simulink model "sampleModel1785_3_sub_sub"  (R2023a)
settings: Solver=VariableStepAuto  StartTime=0.0  StopTime=10.0  RelTol=1e-3
libraries: hdlsllib x4, simulink x2
settings Model: Creator=user1  LastModifiedBy=user1
settings OptimizationCC: BlockReduction=off  ConditionallyExecuteInputs=off

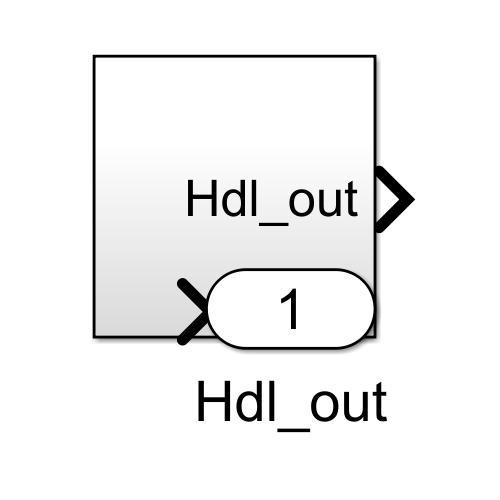
[thumbnail: Simulink's stored preview of the top-level diagram]
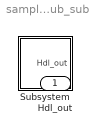
== system sampleModel1785_3_sub_sub ==
  Subsystem : Subsystem
  Hdl_out : Outport  OutDataTypeStr=uint8

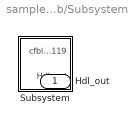
== system sampleModel1785_3_sub_sub/Subsystem ==
  Subsystem : Subsystem
  Hdl_out : Outport  OutDataTypeStr=uint8

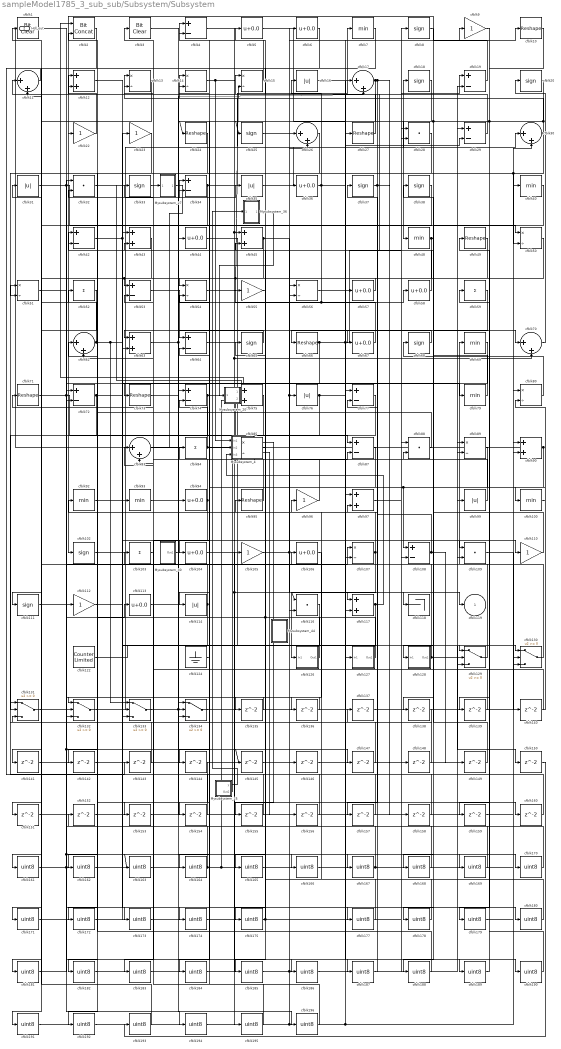
== system sampleModel1785_3_sub_sub/Subsystem/Subsystem ==
  Mysubsystem_20 : Subsystem  TreatAsAtomicUnit=on  RTWFcnName=Mysubsystem_20
      settings: RTWFcnNameOpts=User specified  RTWFileNameOpts=Use function name
  Mysubsystem_25 : Subsystem  TreatAsAtomicUnit=on  RTWFcnName=Mysubsystem_25
      settings: RTWFcnNameOpts=User specified  RTWFileNameOpts=Use function name
  Mysubsystem_27 : Subsystem  TreatAsAtomicUnit=on  RTWFcnName=Mysubsystem_27
      settings: RTWFcnNameOpts=User specified  RTWFileNameOpts=Use function name
  Mysubsystem_30 : Subsystem  TreatAsAtomicUnit=on  RTWFcnName=Mysubsystem_30
      settings: RTWFcnNameOpts=User specified  RTWFileNameOpts=Use function name
  Mysubsystem_36 : Subsystem  TreatAsAtomicUnit=on  RTWFcnName=Mysubsystem_36
      settings: RTWFcnNameOpts=User specified  RTWFileNameOpts=Use function name
  Mysubsystem_4 : Subsystem  TreatAsAtomicUnit=on  RTWFcnName=Mysubsystem_4
      settings: RTWFcnNameOpts=User specified  RTWFileNameOpts=Use function name
  Mysubsystem_44 : Subsystem  TreatAsAtomicUnit=on  RTWFcnName=Mysubsystem_44
      settings: RTWFcnNameOpts=User specified  RTWFileNameOpts=Use function name
  cfblk1 : simulink/Logic and Bit Operations/Bit Clear  iBit=0
      settings: LibrarySourceBlock=|
      | hdlsllib/Logic and Bit
      | Operations/Bit Clear
  cfblk{10,24,27,49,66,71,73,95} (8 alike) : Reshape
  cfblk{7,40,48,69,79,92..93,100} (8 alike) : MinMax  OutDataTypeStr=uint8
  cfblk{8,18,20,25,33,37..38,65,68,102,111} (11 alike) : Signum
  cfblk{52,59,84,103} (4 alike) : Sum  Inputs=+  OutDataTypeStr=uint8
  cfblk{5..6,36,44,57..58,67,94,104,106,113} (11 alike) : Bias  Bias=0.0  SaturateOnIntegerOverflow=off
  cfblk{9,22..23,55,96,105,110,112} (8 alike) : Gain  OutDataTypeStr=uint8
  cfblk{13..15,50..51,54,56,80,85,89,107} (11 alike) : Product  Inputs=*/  OutDataTypeStr=uint8  RndMeth=Zero  SaturateOnIntegerOverflow=on
  cfblk{4,19,29,34,42,53,64,72,74,77,87,108} (12 alike) : Sum  Inputs=+-  OutDataTypeStr=uint8
  cfblk{28,32,88,109,116} (5 alike) : DotProduct  OutDataTypeStr=uint8
  cfblk{11,17,26,30,62,70,83} (7 alike) : Sum  Inputs=|++  OutDataTypeStr=uint8
  cfblk{16,31,35,76,99,114} (6 alike) : Abs  OutDataTypeStr=uint8  SaturateOnIntegerOverflow=off
  cfblk{12,43,45,63,75,90,97,117} (8 alike) : Sum  OutDataTypeStr=uint8
  cfblk118 : Terminator
  cfblk122 : hdlsllib/Sources/Counter Limited  uplimit=7  tsamp=-1
  cfblk124 : Ground
  cfblk126 : Subsystem
      settings: LibrarySourceBlock=|
      | hdlsllib/Ports &
      | Subsystems/Subsystem
  cfblk127 : Subsystem
      settings: LibrarySourceBlock=|
      | hdlsllib/Ports &
      | Subsystems/Subsystem
  cfblk128 : Subsystem
      settings: LibrarySourceBlock=|
      | hdlsllib/Ports &
      | Subsystems/Subsystem
  cfblk{129..134} (6 alike) : Switch  OutDataTypeStr=uint8  SaturateOnIntegerOverflow=off  InputSameDT=off
  cfblk{135..160} (26 alike) : Delay  SampleTime=1
  cfblk{161..175,177..196} (35 alike) : DataTypeConversion  OutDataTypeStr=uint8  SaturateOnIntegerOverflow=off  RndMeth=Floor
  cfblk2 : hdlsllib/Logic and Bit Operations/Bit Concat  numInputs=2
  cfblk3 : simulink/Logic and Bit Operations/Bit Clear  iBit=0
      settings: LibrarySourceBlock=|
      | hdlsllib/Logic and Bit
      | Operations/Bit Clear
  cfblk119 : Outport  OutDataTypeStr=uint8  VectorParamsAs1DForOutWhenUnconnected=off
  Hdl_out : Outport  Port=2  OutDataTypeStr=uint8
  wires:
  Mysubsystem_36/1(Out1) -> Mysubsystem_20/1(In1)
  Mysubsystem_25/1(y) -> Mysubsystem_36/1(In1)
  Mysubsystem_30/1(Out1) -> cfblk134/3
  Mysubsystem_27/1(Out1) -> Mysubsystem_4/2(In2)
  Mysubsystem_20/2(Out2) -> Mysubsystem_27/1(In1)
  Mysubsystem_25/2(Out2) -> cfblk85/1
  Mysubsystem_20/1(Out1) -> cfblk2/1
  Mysubsystem_4/2(Out2) -> cfblk156/1
  Mysubsystem_4/1(Out1) -> cfblk155/1
  cfblk196/1 -> cfblk84/1
  cfblk3/1 -> cfblk196/1
  cfblk195/1 -> cfblk3/1
  cfblk54/1 -> cfblk195/1
  cfblk194/1 -> cfblk17/1, cfblk130/3, cfblk36/1
  cfblk193/1 -> cfblk1/1
  cfblk150/1 -> cfblk193/1
  cfblk192/1 -> cfblk56/2
  cfblk191/1 -> cfblk56/1
  cfblk52/1 -> cfblk191/1
  cfblk190/1 -> cfblk49/1
  cfblk56/1 -> cfblk190/1
  cfblk189/1 -> cfblk59/1
  cfblk188/1 -> cfblk152/1
  cfblk59/1 -> cfblk188/1
  cfblk187/1 -> cfblk77/2
  cfblk186/1 -> cfblk77/1
  cfblk185/1 -> cfblk146/1, cfblk109/2
  cfblk184/1 -> cfblk28/2
  cfblk183/1 -> cfblk28/1
  cfblk182/1 -> cfblk105/1
  cfblk28/1 -> cfblk182/1
  cfblk181/1 -> cfblk112/1
  cfblk13/1 -> cfblk181/1
  cfblk180/1 -> cfblk96/1
  cfblk112/1 -> cfblk180/1
  cfblk179/1 -> cfblk40/1
  cfblk9/1 -> cfblk179/1
  cfblk178/1 -> cfblk137/1
  cfblk40/1 -> cfblk178/1
  cfblk177/1 -> cfblk85/2
  cfblk12/1 -> cfblk177/1
  cfblk175/1 -> cfblk65/1, cfblk88/1
  cfblk174/1 -> cfblk26/2
  cfblk92/1 -> cfblk174/1
  cfblk173/1 -> cfblk26/1
  cfblk172/1 -> cfblk6/1
  cfblk26/1 -> cfblk172/1
  cfblk171/1 -> cfblk93/1
  cfblk170/1 -> cfblk89/1
  cfblk93/1 -> cfblk170/1
  cfblk169/1 -> cfblk83/2
  cfblk153/1 -> cfblk169/1
  cfblk168/1 -> cfblk83/1
  cfblk8/1 -> cfblk168/1
  cfblk167/1 -> cfblk32/1, cfblk29/1
  cfblk166/1 -> cfblk90/2
  cfblk32/1 -> cfblk166/1
  cfblk165/1 -> cfblk90/1
  cfblk55/1 -> cfblk165/1
  cfblk164/1 -> cfblk116/2, cfblk75/2, cfblk2/2
  cfblk163/1 -> cfblk43/2
  cfblk162/1 -> cfblk43/1
  cfblk144/1 -> cfblk162/1
  cfblk161/1 -> cfblk99/1, cfblk173/1
  cfblk160/1 -> cfblk54/2
  cfblk159/1 -> cfblk80/1
  cfblk10/1 -> cfblk159/1
  cfblk158/1 -> cfblk97/2
  cfblk157/1 -> cfblk14/2
  cfblk156/1 -> cfblk131/1
  cfblk155/1 -> cfblk72/1
  cfblk154/1 -> cfblk134/1
  cfblk87/1 -> cfblk154/1
  cfblk152/1 -> cfblk34/2
  cfblk151/1 -> cfblk30/2
  cfblk149/1 -> cfblk88/2
  cfblk148/1 -> cfblk12/2
  cfblk147/1 -> cfblk64/2
  cfblk146/1 -> cfblk19/2
  cfblk145/1 -> cfblk45/2
  cfblk116/1 -> cfblk144/1
  cfblk143/1 -> cfblk51/1
  cfblk11/1 -> cfblk143/1
  cfblk142/1 -> cfblk129/2
  cfblk75/1 -> cfblk142/1
  cfblk141/1 -> cfblk89/2
  cfblk6/1 -> cfblk141/1
  cfblk140/1 -> cfblk74/1
  cfblk109/1 -> cfblk140/1
  cfblk139/1 -> cfblk53/2
  cfblk138/1 -> cfblk131/3
  cfblk137/1 -> cfblk108/2
  cfblk136/1 -> cfblk132/2
  cfblk106/1 -> cfblk136/1
  cfblk135/1 -> cfblk132/1
  cfblk7/1 -> cfblk135/1
  cfblk29/1 -> cfblk12/1
  cfblk38/1 -> cfblk111/1
  cfblk30/1 -> cfblk50/2, cfblk114/1, cfblk24/1, cfblk13/2
  cfblk14/1 -> Mysubsystem_4/1(In1), cfblk45/1, cfblk129/3
  cfblk77/1 -> cfblk185/1
  cfblk4/1 -> cfblk70/2, cfblk109/1
  cfblk85/1 -> cfblk175/1
  cfblk20/1 -> cfblk25/1, cfblk138/1, cfblk139/1
  cfblk49/1 -> cfblk132/3, cfblk55/1
  cfblk107/1 -> cfblk126/1(In1), cfblk92/1
  cfblk42/1 -> cfblk23/1, cfblk147/1
  cfblk33/1 -> cfblk70/1
  cfblk24/1 -> cfblk63/2
  cfblk51/1 -> cfblk163/1, cfblk186/1, cfblk145/1
  cfblk73/1 -> cfblk35/1
  cfblk100/1 -> cfblk80/2
  cfblk95/1 -> cfblk62/2
  cfblk44/1 -> cfblk97/1
  cfblk58/1 -> cfblk13/1
  cfblk90/1 -> cfblk164/1, Hdl_out/1
  cfblk97/1 -> cfblk19/1
  cfblk63/1 -> cfblk94/1, cfblk17/2
  cfblk134/1 -> cfblk100/1
  cfblk50/1 -> cfblk53/1, cfblk151/1
  cfblk37/1 -> cfblk67/1, cfblk148/1
  cfblk62/1 -> cfblk110/1, cfblk133/1, cfblk11/2
  cfblk131/1 -> cfblk113/1
  cfblk23/1 -> cfblk51/2
  cfblk53/1 -> cfblk64/1
  cfblk124/1 -> cfblk4/2
  cfblk70/1 -> cfblk20/1
  cfblk15/1 -> cfblk4/1
  cfblk103/1 -> cfblk33/1
  cfblk88/1 -> cfblk52/1
  cfblk1/1 -> cfblk194/1
  cfblk68/1 -> cfblk66/1
  cfblk48/1 -> cfblk128/1(In1), cfblk171/1
  cfblk79/1 -> cfblk38/1
  cfblk65/1 -> cfblk63/1
  cfblk76/1 -> cfblk27/1, cfblk192/1
  cfblk45/1 -> cfblk76/1, cfblk117/2, cfblk104/1
  cfblk111/1 -> cfblk107/1
  cfblk128/1(Out1) -> cfblk103/1, cfblk150/1
  cfblk83/1 -> cfblk167/1
  cfblk72/1 -> cfblk130/2, cfblk131/2
  cfblk69/1 -> cfblk73/1
  cfblk94/1 -> cfblk71/1, cfblk183/1
  cfblk127/1(Out1) -> cfblk42/2, cfblk95/1
  cfblk57/1 -> cfblk54/1
  cfblk22/1 -> cfblk11/1
  cfblk122/1 -> cfblk130/1
  cfblk16/1 -> cfblk127/1(In1)
  cfblk2/1 -> cfblk22/1
  cfblk102/1 -> cfblk30/1
  cfblk114/1 -> cfblk31/1, cfblk153/1
  cfblk105/1 -> cfblk87/2, cfblk117/1
  cfblk31/1 -> cfblk50/1, cfblk189/1
  cfblk133/1 -> cfblk58/1, cfblk187/1
  cfblk84/1 -> cfblk116/1, cfblk160/1, cfblk74/2
  cfblk35/1 -> cfblk18/1
  cfblk104/1 -> cfblk118/1
  cfblk25/1 -> cfblk9/1
  cfblk67/1 -> cfblk15/2, cfblk16/1
  cfblk96/1 -> cfblk42/1
  cfblk99/1 -> cfblk75/1, cfblk32/2
  cfblk89/1 -> cfblk108/1, cfblk107/2
  cfblk71/1 -> cfblk87/1, cfblk79/1
  cfblk74/1 -> cfblk134/2, cfblk119/1
  cfblk17/1 -> cfblk157/1, cfblk158/1, cfblk184/1
  cfblk126/1(Out1) -> cfblk62/1
  cfblk117/1 -> Mysubsystem_4/3(In3), cfblk133/3
  cfblk5/1 -> cfblk57/1
  cfblk132/1 -> cfblk34/1
  cfblk80/1 -> cfblk68/1
  cfblk113/1 -> cfblk44/1
  cfblk27/1 -> cfblk5/1
  cfblk34/1 -> cfblk7/1, cfblk72/2
  cfblk129/1 -> cfblk69/1
  cfblk19/1 -> cfblk102/1
  cfblk36/1 -> cfblk14/1, cfblk29/2
  cfblk64/1 -> cfblk129/1
  cfblk66/1 -> cfblk8/1, cfblk10/1, cfblk133/2
  cfblk130/1 -> cfblk106/1
  cfblk110/1 -> cfblk15/1
  cfblk18/1 -> cfblk48/1
  cfblk43/1 -> cfblk161/1
  cfblk108/1 -> cfblk37/1, cfblk149/1

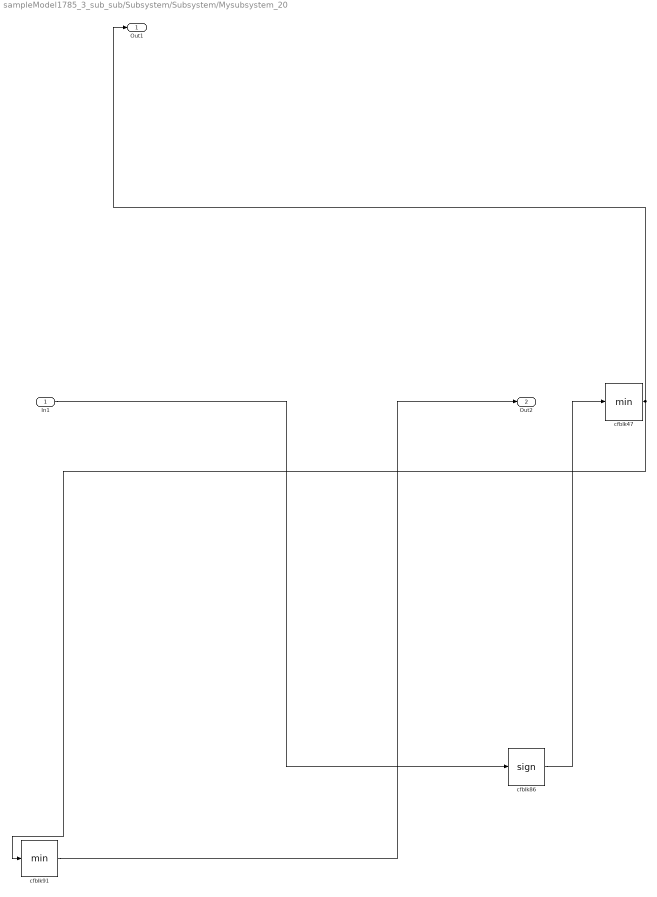
== system sampleModel1785_3_sub_sub/Subsystem/Subsystem/Mysubsystem_20 ==
  In1 : Inport
  cfblk47 : MinMax
  cfblk86 : Signum
  cfblk91 : MinMax
  Out1 : Outport
  Out2 : Outport  Port=2
  wires:
  cfblk86/1 -> cfblk47/1
  cfblk91/1 -> Out2/1
  cfblk47/1 -> Out1/1, cfblk91/1
  In1/1 -> cfblk86/1

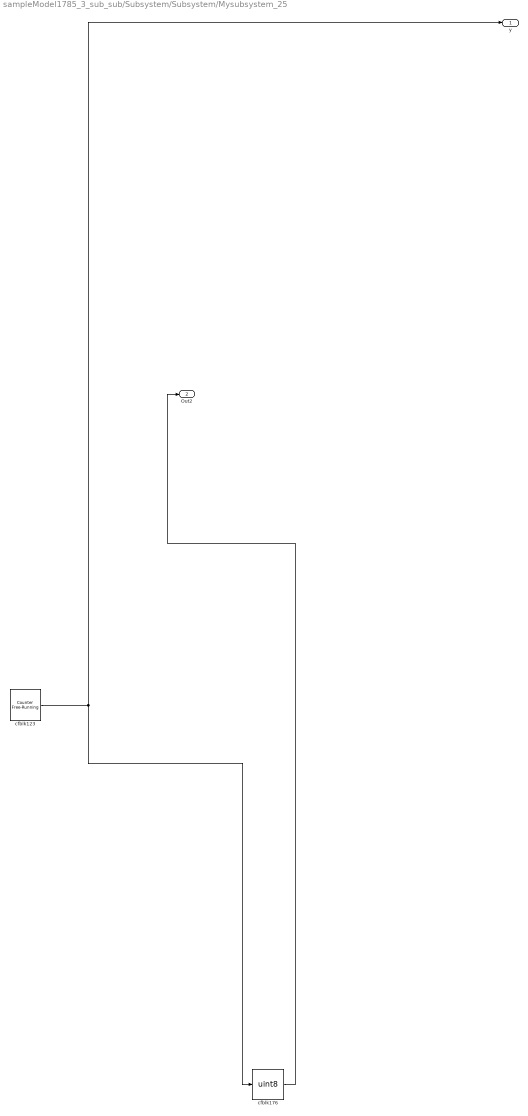
== system sampleModel1785_3_sub_sub/Subsystem/Subsystem/Mysubsystem_25 ==
  cfblk123 : hdlsllib/Sources/Counter Free-Running  NumBits=16  tsamp=-1
  cfblk176 : DataTypeConversion  OutDataTypeStr=uint8  SaturateOnIntegerOverflow=off  RndMeth=Floor
  y : Outport
  Out2 : Outport  Port=2
  wires:
  cfblk123/1 -> y/1, cfblk176/1
  cfblk176/1 -> Out2/1

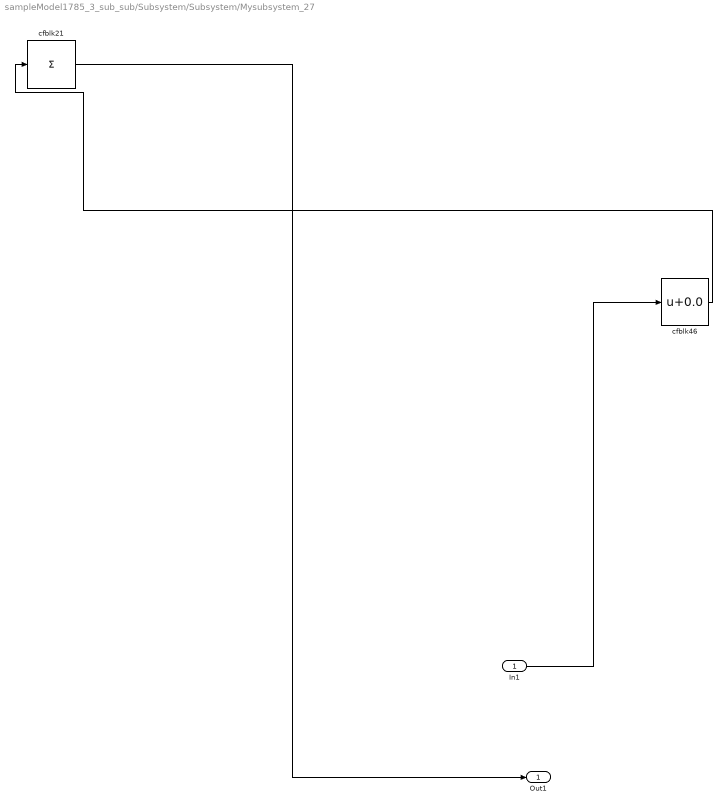
== system sampleModel1785_3_sub_sub/Subsystem/Subsystem/Mysubsystem_27 ==
  In1 : Inport
  cfblk21 : Sum  Inputs=+
  cfblk46 : Bias  Bias=0.0  SaturateOnIntegerOverflow=off
  Out1 : Outport
  wires:
  cfblk21/1 -> Out1/1
  cfblk46/1 -> cfblk21/1
  In1/1 -> cfblk46/1

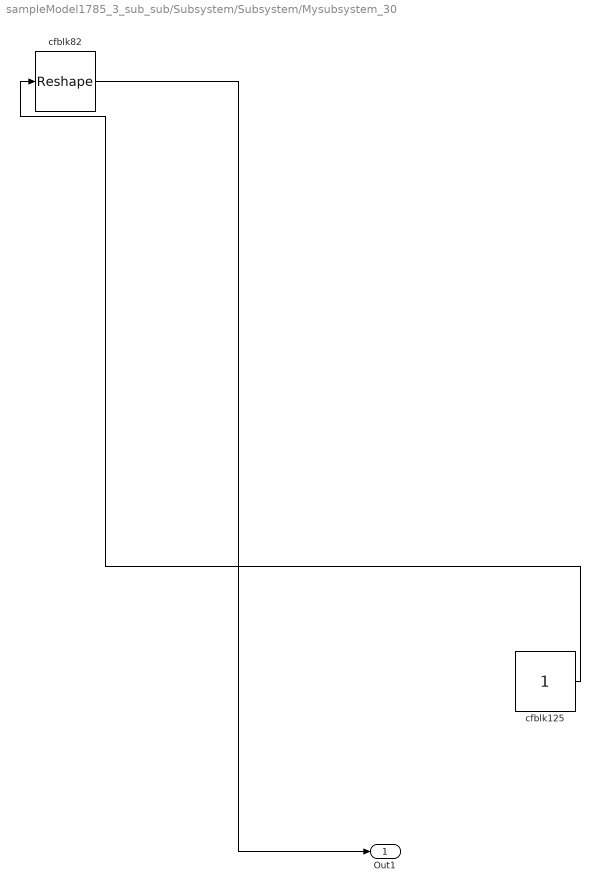
== system sampleModel1785_3_sub_sub/Subsystem/Subsystem/Mysubsystem_30 ==
  cfblk125 : Constant  SampleTime=-1
  cfblk82 : Reshape
  Out1 : Outport
  wires:
  cfblk125/1 -> cfblk82/1
  cfblk82/1 -> Out1/1

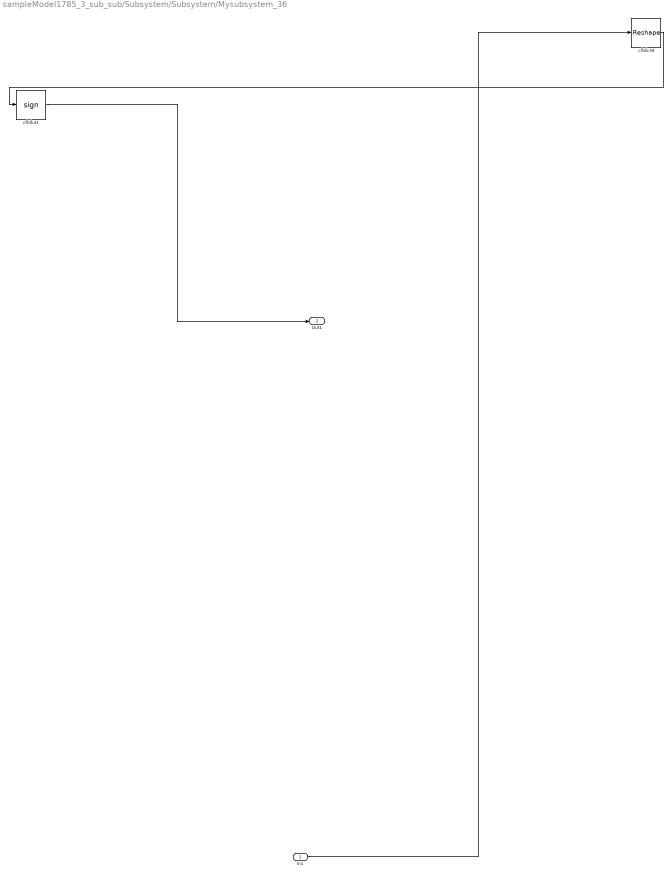
== system sampleModel1785_3_sub_sub/Subsystem/Subsystem/Mysubsystem_36 ==
  In1 : Inport
  cfblk39 : Reshape
  cfblk41 : Signum
  Out1 : Outport
  wires:
  cfblk39/1 -> cfblk41/1
  cfblk41/1 -> Out1/1
  In1/1 -> cfblk39/1

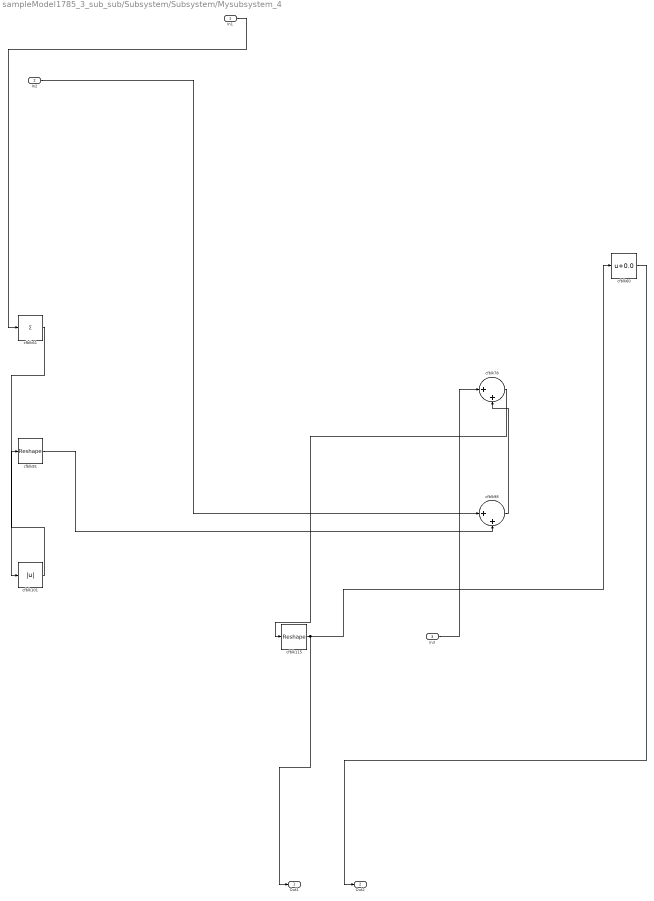
== system sampleModel1785_3_sub_sub/Subsystem/Subsystem/Mysubsystem_4 ==
  In1 : Inport
  In2 : Inport  Port=2
  In3 : Inport  Port=3
  cfblk101 : Abs  SaturateOnIntegerOverflow=off
  cfblk115 : Reshape
  cfblk60 : Bias  Bias=0.0  SaturateOnIntegerOverflow=off
  cfblk61 : Sum  Inputs=+
  cfblk78 : Sum  Inputs=|++
  cfblk81 : Reshape
  cfblk98 : Sum  Inputs=|++
  Out1 : Outport
  Out2 : Outport  Port=2
  wires:
  In1/1 -> cfblk61/1
  cfblk98/1 -> cfblk78/2
  cfblk101/1 -> cfblk81/1
  cfblk61/1 -> cfblk101/1
  cfblk115/1 -> Out1/1, cfblk60/1
  cfblk81/1 -> cfblk98/2
  cfblk60/1 -> Out2/1
  cfblk78/1 -> cfblk115/1
  In3/1 -> cfblk78/1
  In2/1 -> cfblk98/1

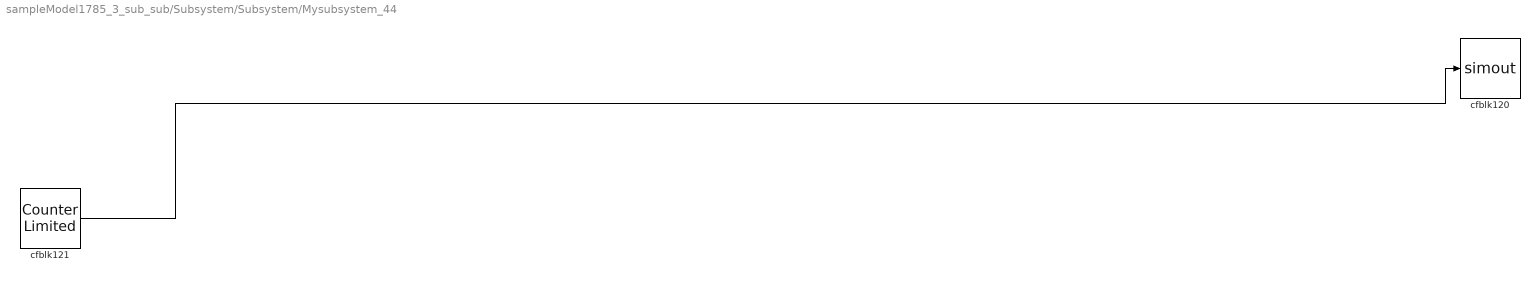
== system sampleModel1785_3_sub_sub/Subsystem/Subsystem/Mysubsystem_44 ==
  cfblk120 : ToWorkspace  VariableName=simout  SaveFormat=Timeseries  SampleTime=-1
  cfblk121 : hdlsllib/Sources/Counter Limited  uplimit=7  tsamp=-1
  wires:
  cfblk121/1 -> cfblk120/1

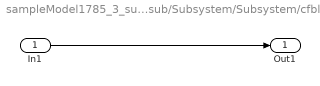
== system sampleModel1785_3_sub_sub/Subsystem/Subsystem/cfblk126 ==
  In1 : Inport
  Out1 : Outport
  wires:
  In1/1 -> Out1/1

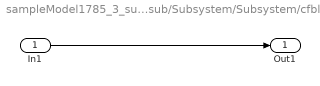
== system sampleModel1785_3_sub_sub/Subsystem/Subsystem/cfblk127 ==
  In1 : Inport
  Out1 : Outport
  wires:
  In1/1 -> Out1/1

== system sampleModel1785_3_sub_sub/Subsystem/Subsystem/cfblk128 ==
  In1 : Inport
  Out1 : Outport
  wires:
  In1/1 -> Out1/1
